simulink model "ThermalElement_Test"  (Simulink 7.7)
settings: Solver=ode45  StartTime=0.0  StopTime=60  RelTol=1e-3
libraries: simulink x1, WZM_QSS_Lib x1
settings Model: Creator=simon  LastModifiedBy=simon

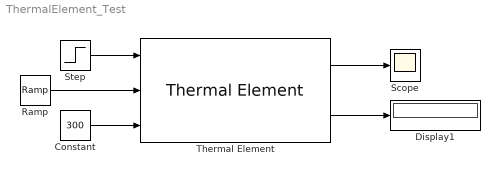
== system ThermalElement_Test ==
  Constant : Constant  Value=300
  Display1 : Display
  Ramp : simulink/Sources/Ramp  SystemSampleTime=-1  slope=20  start=10  X0=0
  Scope : Scope
  Step : Step  Time=5  After=200  SampleTime=0
  Thermal Element : WZM_QSS_Lib/ThermalManagement/Thermal Element  SystemSampleTime=-1  m=200  cp=600  R=0  A=2
  wires:
  Step/1 -> Thermal Element/1
  Ramp/1 -> Thermal Element/2
  Constant/1 -> Thermal Element/3
  Thermal Element/1 -> Scope/1
  Thermal Element/2 -> Display1/1
